simulink model "PLC_Drive_Logic_Rev1_02Mar21"  (R2020b)
settings: Solver=VariableStepAuto  StartTime=0.0  StopTime=Time  MaxStep=0.001  RelTol=1e-3
values from neighbouring files (symbols this model uses):
  Experiment_Start_lookup = [0 0 1 1]    [PLC_setup_Rev1_02Mar21.m]    (also in PLC_setup_Rev3.m; PLC_setup_Rev4.m)
  Experiment_Start_lookup_time = [0 7.680 7.69 8]    [PLC_setup_Rev1_02Mar21.m]    (also in PLC_setup_Rev3.m; PLC_setup_Rev4.m)
  g = 9.81    [PLC_setup_Rev4.m]
  Infeed_r68_Infeed_Current = [8.224174 8.561359 8.023675 12.276806 18.547575 13.840096 19.909491 24.89912 32.847942 30.995712 27.947504 30.215715 ... (6974 elements, 6974x1)]    [Chapter_2_10_Experiment.mat]    (also in Chapter_2_7_Hoisting.mat = [17.475737 19.884655 21.217911 16.409754 16.315434 17.720606; Chapter_2_7_Lowering.mat = [15.937264 23.449905 19.104185 16.13957 17.972174 16.010969 ; PLC_setup_Rev3.m = zeros(1,length(Time_ms)); PLC_setup_Rev4.m = zeros(1,length(Time_ms)))
  Infeed_r70_DC_Voltage = [645.5 644.900024 644.900024 645.700012 645.900024 644.900024 644.700012 644.799988 644.400024 643.5 644.5 644.799988 ... (6974 elements, 6974x1)]    [Chapter_2_10_Experiment.mat]    (also in Chapter_2_7_Hoisting.mat = [644.900024 645 644.900024 644.799988 645.299988 644.900024 ; Chapter_2_7_Lowering.mat = [644.799988 645.200012 644.900024 645.200012 644.900024 644.)
  Infeed_r82_Power_kW = [-2.522412 -4.424248 5.7669 5.876659 12.319849 7.297914 6.612526 10.018862 5.581205 1.580278 3.389305 -1.193998 ... (6974 elements, 6974x1)]    [Chapter_2_10_Experiment.mat]    (also in Chapter_2_7_Hoisting.mat = [2.5658 1.442433 3.361063 1.757025 3.889776 3.03777 4.550285; Chapter_2_7_Lowering.mat = [5.727245 0.282525 2.504848 2.323813 1.020193 5.688412 -2.28)
  mass = 50*10^3    (= 50000)    [PLC_setup_Rev1_02Mar21.m]    (also in PLC_setup_Rev4.m)
  Speed_lookup = [0 0 1000 -1000 500 -500 0 0]    [PLC_setup_Rev1_02Mar21.m]    (also in PLC_setup_Rev3.m; PLC_setup_Rev4.m)
  Speed_lookup_time = [-2 0 2 4 7 10 12 14]+7.14    [PLC_setup_Rev1_02Mar21.m]    (also in PLC_setup_Rev3.m; PLC_setup_Rev4.m)
  Time_ms = [0 4 8 12 16 20 24 28 32 36 40 44 ... (6974 elements, 6974x1)]    [Chapter_2_10_Experiment.mat]    (also in Chapter_2_7_Hoisting.mat = [0 4 8 12 16 20 24 28 32 36 40 44 ... (3041 elements, 3041x1; Chapter_2_7_Lowering.mat = [0 4 8 12 16 20 24 28 32 36 40 44 ... (2736 elements, 2736x1)
  Winch1_r1114_1_SpeedSetpoint = zeros(1,length(Time_ms))    [PLC_setup_Rev1_02Mar21.m]    (also in PLC_setup_Rev3.m; PLC_setup_Rev4.m)
  Winch1_r2060_1_SpeedSetpoint = [1179648 1179648 1179648 1179648 1179648 1179648 1179648 1179648 1179648 1179648 1179648 1179648 ... (6974 elements, 6974x1)]    [Chapter_2_10_Experiment.mat]    (also in Chapter_2_7_Hoisting.mat = [1179648 1179648 1179648 1179648 1179648 1179648 1179648 117; Chapter_2_7_Lowering.mat = [1179648 1179648 1179648 1179648 1179648 1179648 1179648 117; PLC_setup_Rev3.m = zeros(1,length(Time_ms)); PLC_setup_Rev4.m = zeros(1,length(Time_ms)))
  Winch1_r61_Speed = [0 0 0 0 0 0 0 0 0 0 0 0 ... (6974 elements, 6974x1)]    [Chapter_2_10_Experiment.mat]    (also in Chapter_2_7_Hoisting.mat = [0 0 0 0 0 0 0 0 0 0 0 0 ... (3041 elements, 3041x1)]; Chapter_2_7_Lowering.mat = [0 0 0 0 0 0 0 0 0 0 0 0 ... (2736 elements, 2736x1)])
  Winch1_r79_TorqueSetpoint = zeros(1,length(Time_ms))    [PLC_setup_Rev1_02Mar21.m]    (also in PLC_setup_Rev3.m; PLC_setup_Rev4.m)
  Winch1_r80_Torque = [18.736677 17.825405 18.656076 18.489901 18.4027 18.819769 17.939194 18.506048 17.923788 18.604708 18.668221 18.378654 ... (6974 elements, 6974x1)]    [Chapter_2_10_Experiment.mat]    (also in Chapter_2_7_Hoisting.mat = [18.272034 18.472712 18.46044 18.086414 18.336395 18.423048 ; Chapter_2_7_Lowering.mat = [18.344267 18.167727 18.324129 18.318508 18.425446 18.208359)
  Winch2_r61_Speed = [0 0 0 0 0 0 0 0 0 0 0 0 ... (6974 elements, 6974x1)]    [Chapter_2_10_Experiment.mat]    (also in Chapter_2_7_Hoisting.mat = [0 0 0 0 0 0 0 0 0 0 0 0 ... (3041 elements, 3041x1)]; Chapter_2_7_Lowering.mat = [0 0 0 0 0 0 0 0 0 0 0 0 ... (2736 elements, 2736x1)])
  Winch2_r80_Torque = [18.472647 18.501623 18.421309 18.531836 18.286661 18.273392 18.34226 18.525635 18.274195 18.433395 18.206085 18.233738 ... (6974 elements, 6974x1)]    [Chapter_2_10_Experiment.mat]    (also in Chapter_2_7_Hoisting.mat = [18.315447 18.684879 18.200329 18.391209 18.370071 18.122576; Chapter_2_7_Lowering.mat = [18.400066 18.658113 18.092432 18.274298 18.353979 18.215385)
libraries: Control_Library_Rev1_02Mar21 x1
settings Model: Creator=JillMacPherson  LastModifiedBy=Pawel

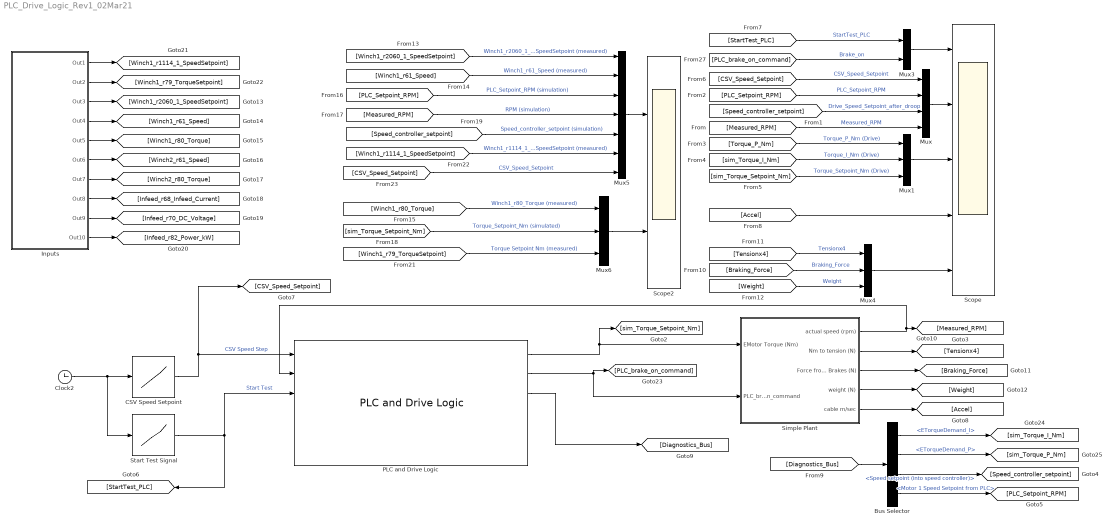
== system PLC_Drive_Logic_Rev1_02Mar21 ==
  Bus Selector : BusSelector  OutputSignals=|
      | ETorqueDemand_I,ETorqueDemand_P,Speed setpoint
      | (into speed controller),Motor 1 Speed Setpoint from PLC
  CSV Speed Setpoint : Lookup_n-D  NumberOfTableDimensions=1  BreakpointsForDimension1=Speed_lookup_time  Table=Speed_lookup  InternalRulePriority=Speed  RndMeth=Simplest  InputSameDT=on
  Clock2 : Clock
  Inputs : Subsystem
  Mux : Mux
  Mux1 : Mux  Inputs=3
  Mux3 : Mux  Inputs=2
  Mux4 : Mux  Inputs=3
  Mux5 : Mux  Inputs=7
  Mux6 : Mux  Inputs=3
  PLC and Drive Logic : Control_Library_Rev1_02Mar21/PLC and Drive Logic  SystemSampleTime=-1  VariantActivationTime=update diagram  Latency=0  AutoFrameSizeCalculation=off
  Scope : Scope  NumInputPorts=5
  Scope2 : Scope  NumInputPorts=2
  Simple Plant : Subsystem
  Start Test Signal : Lookup_n-D  NumberOfTableDimensions=1  BreakpointsForDimension1=Experiment_Start_lookup_time  Table=Experiment_Start_lookup  InternalRulePriority=Speed  RndMeth=Simplest  InputSameDT=on
  wires:
  [Torque_P_Nm] -> Mux1/1  "Torque_P_Nm (Drive)"
  [sim_Torque_I_Nm] -> Mux1/2  "Torque_I_Nm (Drive)"
  [sim_Torque_Setpoint_Nm] -> Mux1/3  "Torque_Setpoint_Nm (Drive)"
  Mux1/1 -> Scope/3
  Mux/1 -> Scope/2
  [StartTest_PLC] -> Mux3/1  "StartTest_PLC"
  Start Test Signal/1 -> PLC and Drive Logic/3, [StartTest_PLC]  "Start Test"
  CSV Speed Setpoint/1 -> PLC and Drive Logic/1, [CSV_Speed_Setpoint]  "CSV Speed Step"
  [Speed_controller_setpoint] -> Mux/3  "Drive_Speed_Setpoint_after_droop"
  [Measured_RPM] -> Mux/4  "Measured_RPM"
  [PLC_Setpoint_RPM] -> Mux/2  "PLC_Setpoint_RPM"
  [CSV_Speed_Setpoint] -> Mux/1  "CSV_Speed_Setpoint"
  [Accel] -> Scope/4
  Mux3/1 -> Scope/1
  [PLC_brake_on_command] -> Mux3/2  "Brake_on"
  [Tensionx4] -> Mux4/1  "Tensionx4"
  [Braking_Force] -> Mux4/2  "Braking_Force"
  Mux4/1 -> Scope/5
  [Weight] -> Mux4/3  "Weight"
  [Winch1_r2060_1_SpeedSetpoint] -> Mux5/1  "Winch1_r2060_1_SpeedSetpoint (measured)"
  [Winch1_r61_Speed] -> Mux5/2  "Winch1_r61_Speed (measured)"
  Mux5/1 -> Scope2/1
  [Winch1_r80_Torque] -> Mux6/1  "Winch1_r80_Torque (measured)"
  Clock2/1 -> Start Test Signal/1, CSV Speed Setpoint/1
  [PLC_Setpoint_RPM] -> Mux5/3  "PLC_Setpoint_RPM (simulation)"
  [Measured_RPM] -> Mux5/4  "RPM (simulation)"
  [sim_Torque_Setpoint_Nm] -> Mux6/2  "Torque_Setpoint_Nm (simulated)"
  Mux6/1 -> Scope2/2
  [Speed_controller_setpoint] -> Mux5/5  "Speed_controller_setpoint (simulation)"
  [Winch1_r1114_1_SpeedSetpoint] -> Mux5/6  "Winch1_r1114_1_SpeedSetpoint (measured)"
  [Winch1_r79_TorqueSetpoint] -> Mux6/3  "Torque Setpoint Nm (measured)"
  Inputs/1(Out1) -> [Winch1_r1114_1_SpeedSetpoint]
  Inputs/2(Out2) -> [Winch1_r79_TorqueSetpoint]
  Inputs/3(Out3) -> [Winch1_r2060_1_SpeedSetpoint]
  Inputs/4(Out4) -> [Winch1_r61_Speed]
  Inputs/5(Out5) -> [Winch1_r80_Torque]
  Inputs/6(Out6) -> [Winch2_r61_Speed]
  Inputs/7(Out7) -> [Winch2_r80_Torque]
  Inputs/8(Out8) -> [Infeed_r68_Infeed_Current]
  Inputs/9(Out9) -> [Infeed_r70_DC_Voltage]
  Inputs/10(Out10) -> [Infeed_r82_Power_kW]
  PLC and Drive Logic/1 -> [sim_Torque_Setpoint_Nm], Simple Plant/1(EMotor Torque (Nm))
  [CSV_Speed_Setpoint] -> Mux5/7  "CSV_Speed_Setpoint"
  Simple Plant/1(actual speed (rpm)) -> PLC and Drive Logic/2, [Measured_RPM]
  PLC and Drive Logic/2 -> Simple Plant/2(PLC_brake_on_command), [PLC_brake_on_command]
  Simple Plant/2(Nm to tension (N)) -> [Tensionx4]
  Simple Plant/3(Force from Brakes (N)) -> [Braking_Force]
  Simple Plant/4(weight (N)) -> [Weight]
  Simple Plant/5(cable m/sec) -> [Accel]
  PLC and Drive Logic/3 -> [Diagnostics_Bus]
  [Diagnostics_Bus] -> Bus Selector/1
  Bus Selector/1 -> [sim_Torque_I_Nm]  "<ETorqueDemand_I>"
  Bus Selector/2 -> [sim_Torque_P_Nm]  "<ETorqueDemand_P>"
  Bus Selector/3 -> [Speed_controller_setpoint]  "<Speed setpoint (into speed controller)>"
  Bus Selector/4 -> [PLC_Setpoint_RPM]  "<Motor 1 Speed Setpoint from PLC>"

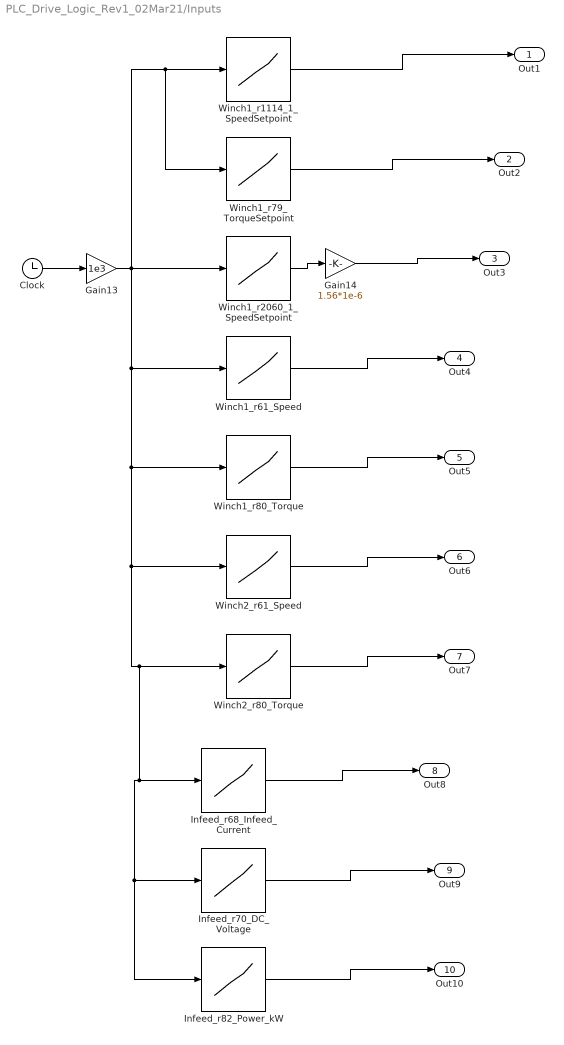
== system PLC_Drive_Logic_Rev1_02Mar21/Inputs ==
  Clock : Clock
  Gain13 : Gain  Gain=1e3
  Gain14 : Gain  Gain=1.56*1e-6
  Infeed_r68_Infeed_Current : Lookup_n-D  NumberOfTableDimensions=1  BreakpointsForDimension1=Time_ms  Table=Infeed_r68_Infeed_Current  InternalRulePriority=Speed  RndMeth=Simplest  InputSameDT=on
  Infeed_r70_DC_Voltage : Lookup_n-D  NumberOfTableDimensions=1  BreakpointsForDimension1=Time_ms  Table=Infeed_r70_DC_Voltage  InternalRulePriority=Speed  RndMeth=Simplest  InputSameDT=on
  Infeed_r82_Power_kW : Lookup_n-D  NumberOfTableDimensions=1  BreakpointsForDimension1=Time_ms  Table=Infeed_r82_Power_kW  InternalRulePriority=Speed  RndMeth=Simplest  InputSameDT=on
  Winch1_r1114_1_SpeedSetpoint : Lookup_n-D  NumberOfTableDimensions=1  BreakpointsForDimension1=Time_ms  Table=Winch1_r1114_1_SpeedSetpoint  InternalRulePriority=Speed  RndMeth=Simplest  InputSameDT=on
  Winch1_r2060_1_SpeedSetpoint : Lookup_n-D  NumberOfTableDimensions=1  BreakpointsForDimension1=Time_ms  Table=Winch1_r2060_1_SpeedSetpoint  InternalRulePriority=Speed  RndMeth=Simplest  InputSameDT=on
  Winch1_r61_Speed : Lookup_n-D  NumberOfTableDimensions=1  BreakpointsForDimension1=Time_ms  Table=Winch1_r61_Speed  InternalRulePriority=Speed  RndMeth=Simplest  InputSameDT=on
  Winch1_r79_TorqueSetpoint : Lookup_n-D  NumberOfTableDimensions=1  BreakpointsForDimension1=Time_ms  Table=Winch1_r79_TorqueSetpoint  InternalRulePriority=Speed  RndMeth=Simplest  InputSameDT=on
  Winch1_r80_Torque : Lookup_n-D  NumberOfTableDimensions=1  BreakpointsForDimension1=Time_ms  Table=Winch1_r80_Torque  InternalRulePriority=Speed  RndMeth=Simplest  InputSameDT=on
  Winch2_r61_Speed : Lookup_n-D  NumberOfTableDimensions=1  BreakpointsForDimension1=Time_ms  Table=Winch2_r61_Speed  InternalRulePriority=Speed  RndMeth=Simplest  InputSameDT=on
  Winch2_r80_Torque : Lookup_n-D  NumberOfTableDimensions=1  BreakpointsForDimension1=Time_ms  Table=Winch2_r80_Torque  InternalRulePriority=Speed  RndMeth=Simplest  InputSameDT=on
  Out1 : Outport
  Out2 : Outport  Port=2
  Out3 : Outport  Port=3
  Out4 : Outport  Port=4
  Out5 : Outport  Port=5
  Out6 : Outport  Port=6
  Out7 : Outport  Port=7
  Out8 : Outport  Port=8
  Out9 : Outport  Port=9
  Out10 : Outport  Port=10
  wires:
  Winch2_r80_Torque/1 -> Out7/1
  Gain14/1 -> Out3/1
  Gain13/1 -> Infeed_r82_Power_kW/1, Infeed_r70_DC_Voltage/1, Infeed_r68_Infeed_Current/1, Winch2_r80_Torque/1, Winch2_r61_Speed/1, Winch1_r80_Torque/1, Winch1_r61_Speed/1, Winch1_r1114_1_SpeedSetpoint/1, Winch1_r79_TorqueSetpoint/1, Winch1_r2060_1_SpeedSetpoint/1
  Winch1_r61_Speed/1 -> Out4/1
  Clock/1 -> Gain13/1
  Infeed_r68_Infeed_Current/1 -> Out8/1
  Winch1_r2060_1_SpeedSetpoint/1 -> Gain14/1
  Winch2_r61_Speed/1 -> Out6/1
  Infeed_r70_DC_Voltage/1 -> Out9/1
  Winch1_r80_Torque/1 -> Out5/1
  Infeed_r82_Power_kW/1 -> Out10/1
  Winch1_r79_TorqueSetpoint/1 -> Out2/1
  Winch1_r1114_1_SpeedSetpoint/1 -> Out1/1

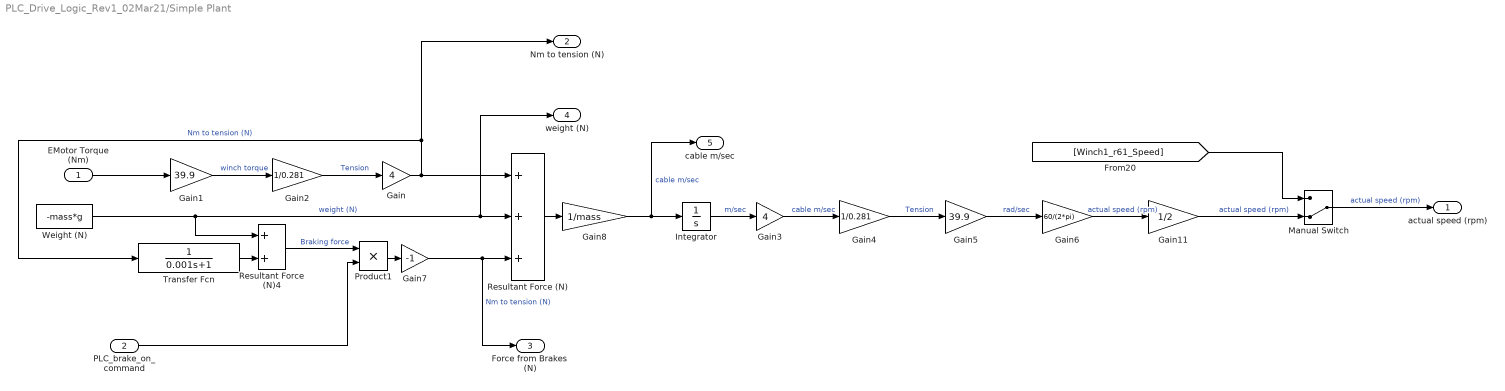
== system PLC_Drive_Logic_Rev1_02Mar21/Simple Plant ==
  EMotor Torque (Nm) : Inport
  PLC_brake_on_command : Inport  Port=2
  Gain : Gain  Gain=4
  Gain1 : Gain  Gain=39.9
  Gain11 : Gain  Gain=1/2
  Gain2 : Gain  Gain=1/0.281
  Gain3 : Gain  Gain=4
  Gain4 : Gain  Gain=1/0.281
  Gain5 : Gain  Gain=39.9
  Gain6 : Gain  Gain=60/(2*pi)
  Gain7 : Gain  Gain=-1
  Gain8 : Gain  Gain=1/mass
  Integrator : Integrator
  Manual Switch : ManualSwitch  CurrentSetting=0
  Product1 : Product
  Resultant Force (N) : Sum  Inputs=+++
  Resultant Force (N)4 : Sum
  Transfer Fcn : TransferFcn  Denominator=[0.001 1]
  Weight (N) : Constant  Value=-mass*g
  actual speed (rpm) : Outport
  Nm to tension (N) : Outport  Port=2
  Force from Brakes (N) : Outport  Port=3
  weight (N) : Outport  Port=4
  cable m/sec : Outport  Port=5
  wires:
  PLC_brake_on_command/1 -> Product1/2
  Manual Switch/1 -> actual speed (rpm)/1  "actual speed (rpm)"
  Integrator/1 -> Gain3/1  "m/sec"
  Gain8/1 -> cable m/sec/1, Integrator/1  "cable m/sec"
  Gain11/1 -> Manual Switch/2  "actual speed (rpm)"
  EMotor Torque (Nm)/1 -> Gain1/1
  Gain3/1 -> Gain4/1  "cable m/sec"
  Gain7/1 -> Resultant Force (N)/3, Force from Brakes (N)/1  "Nm to tension (N)"
  Gain/1 -> Transfer Fcn/1, Nm to tension (N)/1, Resultant Force (N)/1  "Nm to tension (N)"
  Transfer Fcn/1 -> Resultant Force (N)4/2
  Gain4/1 -> Gain5/1  "Tension"
  Weight (N)/1 -> Resultant Force (N)4/1, weight (N)/1, Resultant Force (N)/2  "weight (N)"
  Gain1/1 -> Gain2/1  "winch torque"
  Product1/1 -> Gain7/1
  Gain6/1 -> Gain11/1  "actual speed (rpm)"
  Gain2/1 -> Gain/1  "Tension"
  Resultant Force (N)/1 -> Gain8/1
  Gain5/1 -> Gain6/1  "rad/sec"
  Resultant Force (N)4/1 -> Product1/1  "Braking force"
  [Winch1_r61_Speed] -> Manual Switch/1
